simulink model "PID_ESO_2016b"  (R2016b)
settings: Solver=FixedStepAuto  StartTime=0.0  StopTime=10.0  FixedStep=0.001  RelTol=1e-3
values from neighbouring files (symbols this model uses):
  b0 = 1.5    [Para.m]
  D = 80    [Para.m]
  I = 10    [Para.m]
  k1 = alpha1/epsilon    (= 300)    [Para.m]
  k2 = alpha2/epsilon^2    (= 30000)    [Para.m]
  k3 = alpha3/epsilon^3    (= 1000000)    [Para.m]
  P = 200    [Para.m]
libraries: simulink x2
settings Model: Creator=chengqian  LastModifiedBy=chengqian
settings SFSimCC: SimUseLocalCustomCode=on
settings RTWCC: RTWUseLocalCustomCode=on

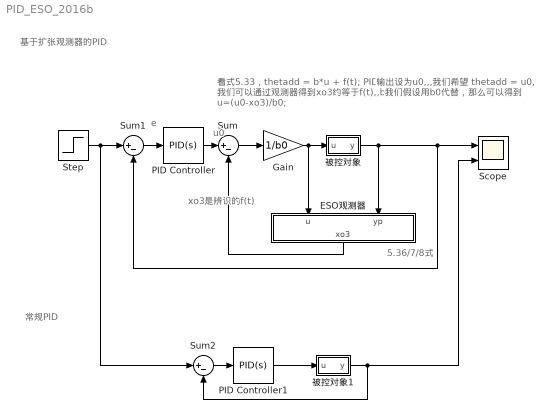
== system PID_ESO_2016b ==
  note: 常规PID
  note: 基于扩张观测器的PID
  note: u0
  note: e
  note: 看式5.33，thetadd = b*u + f(t);
      | PID输出设为u0,,,我们希望 thetadd = u0,
      | 我们可以通过观测器得到xo3约等于f(t),,b我们假设用b0代替，那么可以得到
      | u=(u0-xo3)/b0;
  note: xo3是辨识的f(t)
  note: 5.36/7/8式
  ESO观测器 : Subsystem
  Gain : Gain  Gain=1/b0
  PID Controller : simulink/Continuous/PID Controller  Controller=PID  Form=Parallel  TimeDomain=Continuous-time  SampleTime=-1  IntegratorMethod=Forward Euler  FilterMethod=Forward Euler  ControllerParametersSource=internal  P=P  I=I  D=D  UseFilter=on  N=1000  InitialConditionSource=internal  InitialConditionForIntegrator=0  InitialConditionForFilter=0  DifferentiatorICPrevScaledInput=0  ExternalReset=none  TrackingMode=off  Kt=1  LimitOutput=off  UpperSaturationLimit=inf  LowerSaturationLimit=-inf  LinearizeAsGain=on  AntiWindupMode=none  Kb=1  POutMin=[]  POutMax=[]  IOutMin=[]  IOutMax=[]  DOutMin=[]  DOutMax=[]  NOutMin=[]  NOutMax=[]  SumOutMin=[]  SumOutMax=[]  SaturationOutMin=[]  SaturationOutMax=[]  PParamMin=[]  PParamMax=[]  IParamMin=[]  IParamMax=[]  DParamMin=[]  DParamMax=[]  NParamMin=[]  NParamMax=[]  KbParamMin=[]  KbParamMax=[]  KtParamMin=[]  KtParamMax=[]  KbOutMin=[]  KbOutMax=[]  KtOutMin=[]  KtOutMax=[]  IntegratorOutMin=[]  IntegratorOutMax=[]  FilterOutMin=[]  FilterOutMax=[]  SumI1OutMin=[]  SumI1OutMax=[]  SumI2OutMin=[]  SumI2OutMax=[]  SumI3OutMin=[]  SumI3OutMax=[]  SumDOutMin=[]  SumDOutMax=[]  DifferentiatorOutMin=[]  DifferentiatorOutMax=[]  IntegratorContinuousStateAttributes=''  IntegratorStateMustResolveToSignalObject=off  IntegratorRTWStateStorageClass=Auto  FilterContinuousStateAttributes=''  FilterStateMustResolveToSignalObject=off  FilterRTWStateStorageClass=Auto
  PID Controller1 : simulink/Continuous/PID Controller  Controller=PID  Form=Parallel  TimeDomain=Continuous-time  SampleTime=-1  IntegratorMethod=Forward Euler  FilterMethod=Forward Euler  ControllerParametersSource=internal  P=P  I=I  D=D  UseFilter=on  N=1000  InitialConditionSource=internal  InitialConditionForIntegrator=0  InitialConditionForFilter=0  DifferentiatorICPrevScaledInput=0  ExternalReset=none  TrackingMode=off  Kt=1  LimitOutput=off  UpperSaturationLimit=inf  LowerSaturationLimit=-inf  LinearizeAsGain=on  AntiWindupMode=none  Kb=1  POutMin=[]  POutMax=[]  IOutMin=[]  IOutMax=[]  DOutMin=[]  DOutMax=[]  NOutMin=[]  NOutMax=[]  SumOutMin=[]  SumOutMax=[]  SaturationOutMin=[]  SaturationOutMax=[]  PParamMin=[]  PParamMax=[]  IParamMin=[]  IParamMax=[]  DParamMin=[]  DParamMax=[]  NParamMin=[]  NParamMax=[]  KbParamMin=[]  KbParamMax=[]  KtParamMin=[]  KtParamMax=[]  KbOutMin=[]  KbOutMax=[]  KtOutMin=[]  KtOutMax=[]  IntegratorOutMin=[]  IntegratorOutMax=[]  FilterOutMin=[]  FilterOutMax=[]  SumI1OutMin=[]  SumI1OutMax=[]  SumI2OutMin=[]  SumI2OutMax=[]  SumI3OutMin=[]  SumI3OutMax=[]  SumDOutMin=[]  SumDOutMax=[]  DifferentiatorOutMin=[]  DifferentiatorOutMax=[]  IntegratorContinuousStateAttributes=''  IntegratorStateMustResolveToSignalObject=off  IntegratorRTWStateStorageClass=Auto  FilterContinuousStateAttributes=''  FilterStateMustResolveToSignalObject=off  FilterRTWStateStorageClass=Auto
  Scope : Scope  NumInputPorts=2
  Step : Step  Time=0  SampleTime=0
  Sum : Sum  Inputs=|+-
  Sum1 : Sum  Inputs=|+-
  Sum2 : Sum  Inputs=|+-
  被控对象 : Subsystem
  被控对象1 : Subsystem
  wires:
  被控对象/1(y) -> Sum1/2, Scope/1, ESO观测器/2(yp)
  PID Controller/1 -> Sum/1
  Sum/1 -> Gain/1
  ESO观测器/1(xo3) -> Sum/2
  Gain/1 -> 被控对象/1(u), ESO观测器/1(u)
  Sum1/1 -> PID Controller/1
  Step/1 -> Sum2/1, Sum1/1
  PID Controller1/1 -> 被控对象1/1(u)
  Sum2/1 -> PID Controller1/1
  被控对象1/1(y) -> Sum2/2, Scope/2

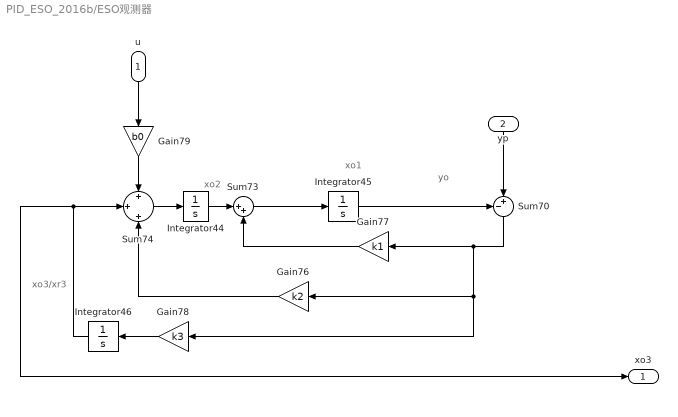
== system PID_ESO_2016b/ESO观测器 ==
  note: xo3/xr3
  note: xo2
  note: xo1
  note: yo
  u : Inport
  yp : Inport  Port=2
  Gain76 : Gain  Gain=k2
  Gain77 : Gain  Gain=k1
  Gain78 : Gain  Gain=k3
  Gain79 : Gain  Gain=b0
  Integrator44 : Integrator
  Integrator45 : Integrator
  Integrator46 : Integrator
  Sum70 : Sum  Inputs=-+|
  Sum73 : Sum  Inputs=|++
  Sum74 : Sum  Inputs=+|+|+
  xo3 : Outport
  wires:
  Integrator46/1 -> Sum74/2, xo3/1
  Sum70/1 -> Gain78/1, Gain76/1, Gain77/1
  Integrator45/1 -> Sum70/1
  Sum74/1 -> Integrator44/1
  Gain78/1 -> Integrator46/1
  Gain76/1 -> Sum74/3
  Gain79/1 -> Sum74/1
  yp/1 -> Sum70/2
  u/1 -> Gain79/1
  Sum73/1 -> Integrator45/1
  Integrator44/1 -> Sum73/1
  Gain77/1 -> Sum73/2

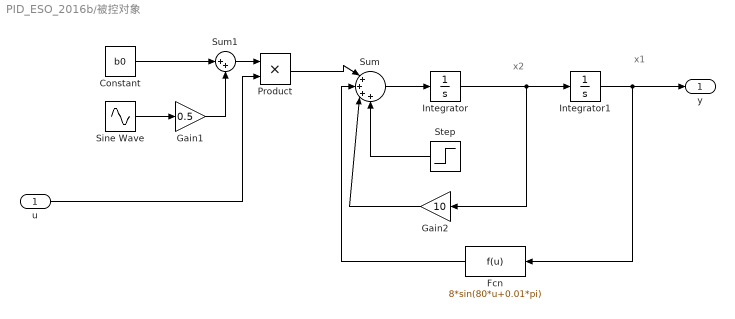
== system PID_ESO_2016b/被控对象 ==
  note: x2
  note: x1
  u : Inport
  Constant : Constant  Value=b0
  Fcn : Fcn  Expr=8*sin(80*u+0.01*pi)
  Gain1 : Gain  Gain=0.5
  Gain2 : Gain  Gain=10
  Integrator : Integrator
  Integrator1 : Integrator
  Product : Product
  Sine Wave : Sin  Bias=1  Frequency=0.2*pi  SampleTime=0
  Step : Step  Time=5  After=100  SampleTime=0
  Sum : Sum  Inputs=|++++
  Sum1 : Sum  Inputs=|++
  y : Outport
  wires:
  Fcn/1 -> Sum/2
  Gain2/1 -> Sum/3
  Product/1 -> Sum/1
  Sine Wave/1 -> Gain1/1
  Sum1/1 -> Product/1
  Gain1/1 -> Sum1/2
  Integrator/1 -> Integrator1/1, Gain2/1
  Constant/1 -> Sum1/1
  u/1 -> Product/2
  Integrator1/1 -> y/1, Fcn/1
  Sum/1 -> Integrator/1
  Step/1 -> Sum/4

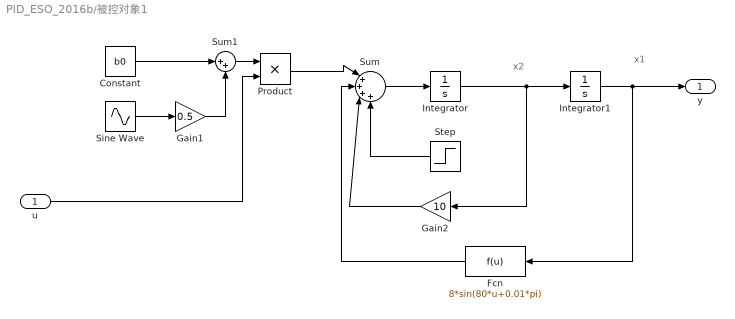
== system PID_ESO_2016b/被控对象1 ==
  note: x2
  note: x1
  u : Inport
  Constant : Constant  Value=b0
  Fcn : Fcn  Expr=8*sin(80*u+0.01*pi)
  Gain1 : Gain  Gain=0.5
  Gain2 : Gain  Gain=10
  Integrator : Integrator
  Integrator1 : Integrator
  Product : Product
  Sine Wave : Sin  Bias=1  Frequency=0.2*pi  SampleTime=0
  Step : Step  Time=5  After=100  SampleTime=0
  Sum : Sum  Inputs=|++++
  Sum1 : Sum  Inputs=|++
  y : Outport
  wires:
  Fcn/1 -> Sum/2
  Gain2/1 -> Sum/3
  Product/1 -> Sum/1
  Sine Wave/1 -> Gain1/1
  Sum1/1 -> Product/1
  Gain1/1 -> Sum1/2
  Integrator/1 -> Integrator1/1, Gain2/1
  Constant/1 -> Sum1/1
  u/1 -> Product/2
  Integrator1/1 -> y/1, Fcn/1
  Sum/1 -> Integrator/1
  Step/1 -> Sum/4
